simulink model "HSM_4p6U10_Motion_v01_06022022_NEW_ECC_2019a"  (R2019a)
settings: Solver=ode1  StartTime=0.0  StopTime=Inf  FixedStep=Ts  RelTol=1e-3  EnableMultiTasking=on
PostLoadFcn:
  | , if any(exist('dsrtsu_mdlpostloadfcn', 'file') == [2, 3, 6]), try dsrtsu_mdlpostloadfcn('Execute', bdroot); catch fprintf('Error in PostLoadFcn (dsrtsu_mdlpostloadfcn) for model "%s":\n %s\n', bdroot, lasterr); end, end,
values from neighbouring files (symbols this model uses):
  CDP = -1    [Parameters_4p6U10.m]
  CUP = 1    [Parameters_4p6U10.m]
  HDP = 1    [Parameters_4p6U10.m]
  HUP = -1    [Parameters_4p6U10.m]
  K1m = 1.7E-4    (= 0.00017)    [Parameters_4p6U10.m]
  K2m = 7.0E-4    (= 0.0007)    [Parameters_4p6U10.m]
  Ts = 0.0002    [Parameters_4p6U10.m]
undefined symbols (not defined in the file or in its folder): GPTRIP1SEL, GPTRIP2SEL, TZ1, TZ2
libraries: simulink_extras x25, simulink x17, c2837xDlib x11, c2802xlib x2, idelinklib_common x1
(part 3 of 3)

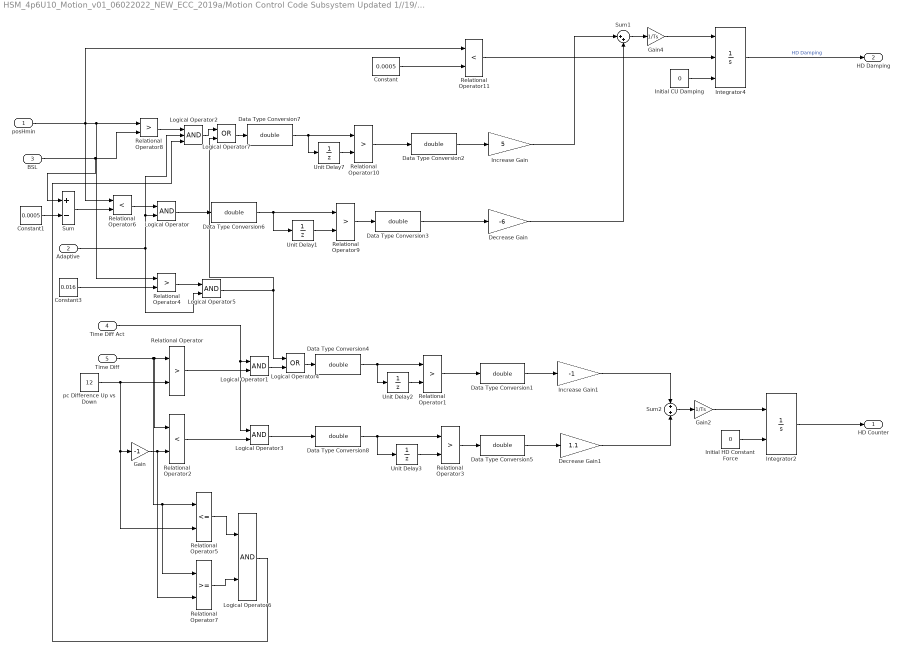
== system HSM_4p6U10_Motion_v01_06022022_NEW_ECC_2019a/Motion Control Code Subsystem Updated 1//19//21/Oscillation, Start Motion, 4 Phases Subsystem/Oscillations Subsystem Time pc No Cold Damping/Subsystem/Approximate Resonance Actuation/Subsystem ==
  posHmin : Inport
  Adaptive : Inport  Port=2
  BSL : Inport  Port=3
  Time Diff Act : Inport  Port=4
  Time Diff : Inport  Port=5
  Constant : Constant  Value=0.0005
  Constant1 : Constant  Value=0.0005
  Constant3 : Constant  Value=0.016
  Data Type Conversion{1..8} (8 alike) : DataTypeConversion  OutDataTypeStr=double
  Decrease Gain : Gain  Gain=-6  OutDataTypeStr=double
  Decrease Gain1 : Gain  Gain=1.1  OutDataTypeStr=double
  Gain : Gain  Gain=-1
  Gain2 : Gain  Gain=1/Ts
  Gain4 : Gain  Gain=1/Ts
  Increase Gain : Gain  Gain=5  OutDataTypeStr=double
  Increase Gain1 : Gain  Gain=-1  OutDataTypeStr=double
  Initial CU Damping : Constant  Value=0  OutDataTypeStr=double
  Initial HD Constant Force : Constant  Value=0  OutDataTypeStr=double
  Integrator2 : Integrator  InitialConditionSource=external  LimitOutput=on  UpperSaturationLimit=2000  LowerSaturationLimit=-2000
  Integrator4 : Integrator  ExternalReset=either  InitialConditionSource=external  LimitOutput=on  UpperSaturationLimit=2000  LowerSaturationLimit=0
  Logical Operator{,1,3,5..6} (5 alike) : Logic  AllPortsSameDT=off  OutDataTypeStr=boolean
  Logical Operator2 : Logic  Inputs=3  AllPortsSameDT=off  OutDataTypeStr=boolean
  Logical Operator4 : Logic  Operator=OR  AllPortsSameDT=off  OutDataTypeStr=boolean
  Logical Operator7 : Logic  Operator=OR  AllPortsSameDT=off  OutDataTypeStr=boolean
  Relational Operator{,1,3..4,8..10} (7 alike) : RelationalOperator  Operator=>  OutDataTypeStr=boolean  RndMeth=Simplest
  Relational Operator11 : RelationalOperator  Operator=<  OutDataTypeStr=boolean  RndMeth=Simplest
  Relational Operator2 : RelationalOperator  Operator=<  OutDataTypeStr=boolean  RndMeth=Simplest
  Relational Operator5 : RelationalOperator  Operator=<=  OutDataTypeStr=boolean  RndMeth=Simplest
  Relational Operator6 : RelationalOperator  Operator=<  OutDataTypeStr=boolean  RndMeth=Simplest
  Relational Operator7 : RelationalOperator  OutDataTypeStr=boolean  RndMeth=Simplest
  Sum : Sum  Inputs=+-
  Sum1 : Sum  Inputs=|++
  Sum2 : Sum
  Unit Delay{1..3,7} (4 alike) : UnitDelay  SampleTime=-1  HasFrameUpgradeWarning=on
  pc Difference Up vs Down : Constant  Value=12
  "HD Counter " : Outport
  HD Damping : Outport  Port=2
  wires:
  BSL/1 -> Relational Operator8/2, Sum/1
  Relational Operator8/1 -> Logical Operator2/1
  Initial CU Damping/1 -> Integrator4/3
  Data Type Conversion6/1 -> Unit Delay1/1, Relational Operator9/1
  Gain4/1 -> Integrator4/1
  Integrator2/1 -> "HD Counter "/1
  Increase Gain/1 -> Sum1/1
  Integrator4/1 -> HD Damping/1  "HD Damping"
  Data Type Conversion7/1 -> Relational Operator10/1, Unit Delay7/1
  Relational Operator10/1 -> Data Type Conversion2/1
  Sum1/1 -> Gain4/1
  posHmin/1 -> Relational Operator6/1, Relational Operator11/1, Relational Operator4/1, Relational Operator8/1
  Logical Operator2/1 -> Logical Operator7/1
  Decrease Gain1/1 -> Sum2/2
  Logical Operator/1 -> Data Type Conversion6/1
  Data Type Conversion2/1 -> Increase Gain/1
  Constant/1 -> Relational Operator11/2
  Unit Delay1/1 -> Relational Operator9/2
  Relational Operator6/1 -> Logical Operator/1
  Sum2/1 -> Gain2/1
  Relational Operator11/1 -> Integrator4/2
  Data Type Conversion3/1 -> Decrease Gain/1
  Increase Gain1/1 -> Sum2/1
  Constant1/1 -> Sum/2
  Adaptive/1 -> Logical Operator2/2, Logical Operator/2, Logical Operator5/2
  Unit Delay7/1 -> Relational Operator10/2
  Sum/1 -> Relational Operator6/2
  Gain2/1 -> Integrator2/1
  Initial HD Constant Force/1 -> Integrator2/2
  Relational Operator9/1 -> Data Type Conversion3/1
  Decrease Gain/1 -> Sum1/2
  Time Diff/1 -> Relational Operator5/1, Relational Operator7/1, Relational Operator2/1, Relational Operator/1
  pc Difference Up vs Down/1 -> Relational Operator/2, Gain/1, Relational Operator5/2
  Relational Operator/1 -> Logical Operator1/2
  Time Diff Act/1 -> Logical Operator1/1, Logical Operator3/1
  Unit Delay2/1 -> Relational Operator1/2
  Data Type Conversion1/1 -> Increase Gain1/1
  Relational Operator1/1 -> Data Type Conversion1/1
  Data Type Conversion4/1 -> Unit Delay2/1, Relational Operator1/1
  Logical Operator1/1 -> Logical Operator4/2
  Gain/1 -> Relational Operator7/2, Relational Operator2/2
  Relational Operator2/1 -> Logical Operator3/2
  Relational Operator3/1 -> Data Type Conversion5/1
  Data Type Conversion5/1 -> Decrease Gain1/1
  Unit Delay3/1 -> Relational Operator3/2
  Data Type Conversion8/1 -> Relational Operator3/1, Unit Delay3/1
  Logical Operator3/1 -> Data Type Conversion8/1
  Logical Operator4/1 -> Data Type Conversion4/1
  Relational Operator4/1 -> Logical Operator5/1
  Constant3/1 -> Relational Operator4/2
  Logical Operator5/1 -> Logical Operator7/2, Logical Operator4/1
  Relational Operator5/1 -> Logical Operator6/1
  Relational Operator7/1 -> Logical Operator6/2
  Logical Operator6/1 -> Logical Operator2/3
  Logical Operator7/1 -> Data Type Conversion7/1

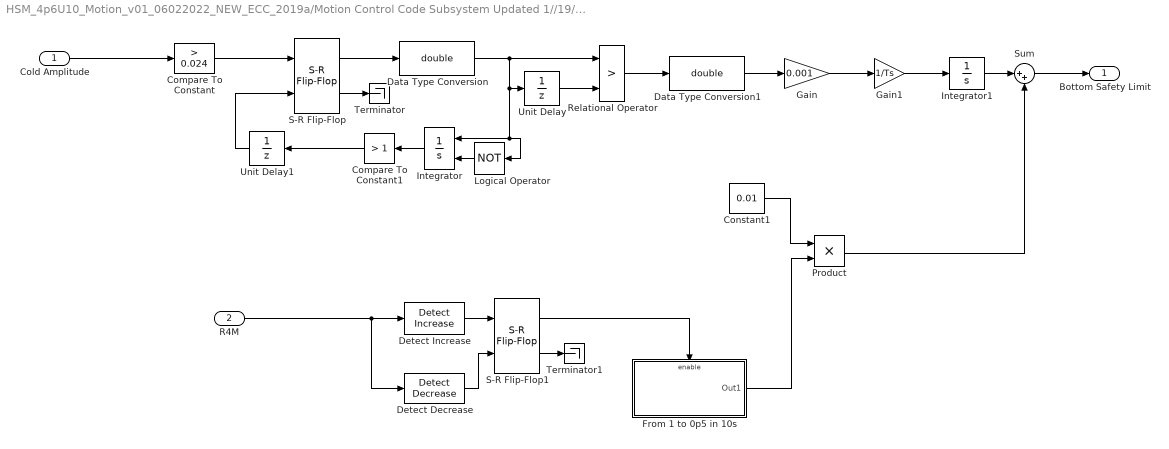
== system HSM_4p6U10_Motion_v01_06022022_NEW_ECC_2019a/Motion Control Code Subsystem Updated 1//19//21/Oscillation, Start Motion, 4 Phases Subsystem/Oscillations Subsystem Time pc No Cold Damping/Subsystem/Approximate Resonance Actuation/Subsystem1 ==
  Cold Amplitude : Inport
  R4M : Inport  Port=2
  Compare To Constant : simulink/Logic and Bit Operations/Compare To Constant  relop=>  const=0.024  OutDataTypeStr=boolean
  Compare To Constant1 : simulink/Logic and Bit Operations/Compare To Constant  relop=>  const=1  OutDataTypeStr=boolean
  Constant1 : Constant  Value=0.01
  Data Type Conversion : DataTypeConversion  OutDataTypeStr=double
  Data Type Conversion1 : DataTypeConversion  OutDataTypeStr=double
  Detect Decrease : simulink/Logic and Bit Operations/Detect Decrease  vinit=0.0  OutDataTypeStr=boolean
  Detect Increase : simulink/Logic and Bit Operations/Detect Increase  vinit=0.0  OutDataTypeStr=boolean
  From 1 to 0p5 in 10s : Subsystem
  Gain : Gain  Gain=0.001
  Gain1 : Gain  Gain=1/Ts
  Integrator : Integrator  ExternalReset=rising
  Integrator1 : Integrator  LimitOutput=on  UpperSaturationLimit=0.006  LowerSaturationLimit=0
  Logical Operator : Logic  Operator=NOT  AllPortsSameDT=off  OutDataTypeStr=boolean
  Product : Product
  Relational Operator : RelationalOperator  Operator=>  OutDataTypeStr=boolean  RndMeth=Simplest
  S-R Flip-Flop : simulink_extras/Flip Flops/S-R Flip-Flop  initial_condition=0
  S-R Flip-Flop1 : simulink_extras/Flip Flops/S-R Flip-Flop  initial_condition=0
  Sum : Sum  Inputs=|++
  Terminator : Terminator
  Terminator1 : Terminator
  Unit Delay : UnitDelay  SampleTime=-1  HasFrameUpgradeWarning=on
  Unit Delay1 : UnitDelay  SampleTime=-1  HasFrameUpgradeWarning=on
  Bottom Safety Limit : Outport
  wires:
  Sum/1 -> Bottom Safety Limit/1
  Integrator1/1 -> Sum/1
  Gain1/1 -> Integrator1/1
  Gain/1 -> Gain1/1
  Unit Delay1/1 -> S-R Flip-Flop/2
  Compare To Constant1/1 -> Unit Delay1/1
  Integrator/1 -> Compare To Constant1/1
  Logical Operator/1 -> Integrator/2
  Data Type Conversion1/1 -> Gain/1
  Relational Operator/1 -> Data Type Conversion1/1
  Unit Delay/1 -> Relational Operator/2
  Data Type Conversion/1 -> Relational Operator/1, Unit Delay/1, Integrator/1, Logical Operator/1
  S-R Flip-Flop/1 -> Data Type Conversion/1
  S-R Flip-Flop/2 -> Terminator/1
  Compare To Constant/1 -> S-R Flip-Flop/1
  Cold Amplitude/1 -> Compare To Constant/1
  Product/1 -> Sum/2
  From 1 to 0p5 in 10s/1(Out1) -> Product/2
  S-R Flip-Flop1/2 -> Terminator1/1
  R4M/1 -> Detect Decrease/1, Detect Increase/1
  S-R Flip-Flop1/1 -> From 1 to 0p5 in 10s/Enable
  Detect Decrease/1 -> S-R Flip-Flop1/2
  Detect Increase/1 -> S-R Flip-Flop1/1
  Constant1/1 -> Product/1

== system HSM_4p6U10_Motion_v01_06022022_NEW_ECC_2019a/Motion Control Code Subsystem Updated 1//19//21/Oscillation, Start Motion, 4 Phases Subsystem/Oscillations Subsystem Time pc No Cold Damping/Subsystem/Approximate Resonance Actuation/Subsystem2 ==
  PosH : Inport
  VelH : Inport  Port=2
  Bot Safety Limit : Inport  Port=3
  posHFRTime : Inport  Port=4
  AND1 : Logic  AllPortsSameDT=off  OutDataTypeStr=boolean
  Constant3 : Constant  Value=0
  Constant5 : Constant  Value=0
  HD Act : simulink_extras/Flip Flops/S-R Flip-Flop  initial_condition=0
  Logical Operator1 : Logic  Operator=OR  AllPortsSameDT=off  OutDataTypeStr=boolean
  OR1 : Logic  Operator=OR  AllPortsSameDT=off  OutDataTypeStr=boolean
  Relational Operator5 : RelationalOperator  Operator=<=  OutDataTypeStr=boolean  RndMeth=Simplest
  Relational Operator6 : RelationalOperator  Operator=>  OutDataTypeStr=boolean  RndMeth=Simplest
  Relational Operator8 : RelationalOperator  Operator=<  OutDataTypeStr=boolean  RndMeth=Simplest
  Relational Operator9 : RelationalOperator  Operator=<  OutDataTypeStr=boolean  RndMeth=Simplest
  Start Hot Down : Constant  Value=0.035
  Subsystem : Subsystem
  Terminator : Terminator
  Unit Delay : UnitDelay  SampleTime=-1  HasFrameUpgradeWarning=on
  HD Activation : Outport
  wires:
  Unit Delay/1 -> HD Act/2
  Logical Operator1/1 -> Unit Delay/1
  HD Act/2 -> Terminator/1
  HD Act/1 -> Subsystem/2(Q Boolean), HD Activation/1  "HD Act"
  Relational Operator6/1 -> OR1/2  "VelH > 0"
  Constant3/1 -> Relational Operator6/2
  Relational Operator5/1 -> OR1/1  "PosH <= Bot Safety"
  Bot Safety Limit/1 -> Relational Operator5/2
  PosH/1 -> Subsystem/3(posH), Relational Operator8/1, Relational Operator5/1
  Constant5/1 -> Relational Operator9/2
  Relational Operator9/1 -> AND1/2  "VelH   < 0"
  Relational Operator8/1 -> AND1/1  "PosH  < 0.025"
  AND1/1 -> HD Act/1
  Start Hot Down/1 -> Relational Operator8/2
  VelH/1 -> Relational Operator9/1, Relational Operator6/1
  OR1/1 -> Logical Operator1/1
  posHFRTime/1 -> Subsystem/1(posHFRTime)
  Subsystem/1(Reset) -> Logical Operator1/2

== system HSM_4p6U10_Motion_v01_06022022_NEW_ECC_2019a/Motion Control Code Subsystem Updated 1//19//21/Oscillation, Start Motion, 4 Phases Subsystem/Oscillations Subsystem Time pc No Cold Damping/Subsystem/Hot Down Control/Unity Gain Scaling ==
  u : Inport
  x : Inport  Port=2
  Constant6 : Constant  Value=K2m
  Gain1 : Gain  Gain=-1/K1m
  IYC Saturation : Saturate  UpperLimit=3600  LowerLimit=0
  Math Function4 : Math  Operator=square  SaturateOnIntegerOverflow=on
  Product1 : Product
  Sqrt : Sqrt  SaturateOnIntegerOverflow=on
  Sum3 : Sum
  i : Outport
  wires:
  IYC Saturation/1 -> Sqrt/1
  Sqrt/1 -> i/1
  Product1/1 -> IYC Saturation/1
  Gain1/1 -> Product1/1
  x/1 -> Sum3/2
  Math Function4/1 -> Product1/2
  Constant6/1 -> Sum3/1
  Sum3/1 -> Math Function4/1
  u/1 -> Gain1/1

== system HSM_4p6U10_Motion_v01_06022022_NEW_ECC_2019a/Motion Control Code Subsystem Updated 1//19//21/Oscillation, Start Motion, 4 Phases Subsystem/Oscillations Subsystem Time pc No Cold Damping/Cold Resonance/Approximate Resonance Actuation/CD Damping/Subsystem ==
  In1 : Inport
  Data Type Conversion1 : DataTypeConversion  OutDataTypeStr=double
  Data Type Conversion2 : DataTypeConversion  OutDataTypeStr=double
  Relational Operator4 : RelationalOperator  Operator=>  OutDataTypeStr=boolean  RndMeth=Simplest
  Unit Delay2 : UnitDelay  SampleTime=-1  HasFrameUpgradeWarning=on
  Out1 : Outport
  wires:
  Relational Operator4/1 -> Data Type Conversion2/1
  Data Type Conversion2/1 -> Out1/1
  Data Type Conversion1/1 -> Relational Operator4/1, Unit Delay2/1
  Unit Delay2/1 -> Relational Operator4/2
  In1/1 -> Data Type Conversion1/1

== system HSM_4p6U10_Motion_v01_06022022_NEW_ECC_2019a/Motion Control Code Subsystem Updated 1//19//21/Oscillation, Start Motion, 4 Phases Subsystem/Oscillations Subsystem Time pc No Cold Damping/Cold Resonance/Approximate Resonance Actuation/CD Damping/Subsystem1 ==
  In1 : Inport
  Data Type Conversion3 : DataTypeConversion  OutDataTypeStr=double
  Data Type Conversion4 : DataTypeConversion  OutDataTypeStr=double
  Relational Operator5 : RelationalOperator  Operator=>  OutDataTypeStr=boolean  RndMeth=Simplest
  Unit Delay1 : UnitDelay  SampleTime=-1  HasFrameUpgradeWarning=on
  Out1 : Outport
  wires:
  Data Type Conversion4/1 -> Out1/1
  Unit Delay1/1 -> Relational Operator5/2
  Relational Operator5/1 -> Data Type Conversion4/1
  In1/1 -> Data Type Conversion3/1
  Data Type Conversion3/1 -> Unit Delay1/1, Relational Operator5/1

== system HSM_4p6U10_Motion_v01_06022022_NEW_ECC_2019a/Motion Control Code Subsystem Updated 1//19//21/Oscillation, Start Motion, 4 Phases Subsystem/Oscillations Subsystem Time pc No Cold Damping/Cold Resonance/Approximate Resonance Actuation/CD Damping/Subsystem2 ==
  In1 : Inport
  Data Type Conversion3 : DataTypeConversion  OutDataTypeStr=double
  Data Type Conversion4 : DataTypeConversion  OutDataTypeStr=double
  Relational Operator5 : RelationalOperator  Operator=>  OutDataTypeStr=boolean  RndMeth=Simplest
  Unit Delay1 : UnitDelay  SampleTime=-1  HasFrameUpgradeWarning=on
  Out1 : Outport
  wires:
  Data Type Conversion3/1 -> Relational Operator5/1, Unit Delay1/1
  In1/1 -> Data Type Conversion3/1
  Relational Operator5/1 -> Data Type Conversion4/1
  Unit Delay1/1 -> Relational Operator5/2
  Data Type Conversion4/1 -> Out1/1

== system HSM_4p6U10_Motion_v01_06022022_NEW_ECC_2019a/Motion Control Code Subsystem Updated 1//19//21/Oscillation, Start Motion, 4 Phases Subsystem/Oscillations Subsystem Time pc No Cold Damping/Cold Resonance/Approximate Resonance Actuation/CD Damping/Subsystem3 ==
  In1 : Inport
  Data Type Conversion3 : DataTypeConversion  OutDataTypeStr=double
  Data Type Conversion4 : DataTypeConversion  OutDataTypeStr=double
  Relational Operator5 : RelationalOperator  Operator=>  OutDataTypeStr=boolean  RndMeth=Simplest
  Unit Delay1 : UnitDelay  SampleTime=-1  HasFrameUpgradeWarning=on
  Out1 : Outport
  wires:
  Data Type Conversion4/1 -> Out1/1
  Unit Delay1/1 -> Relational Operator5/2
  Relational Operator5/1 -> Data Type Conversion4/1
  In1/1 -> Data Type Conversion3/1
  Data Type Conversion3/1 -> Unit Delay1/1, Relational Operator5/1

== system HSM_4p6U10_Motion_v01_06022022_NEW_ECC_2019a/Motion Control Code Subsystem Updated 1//19//21/Oscillation, Start Motion, 4 Phases Subsystem/Oscillations Subsystem Time pc No Cold Damping/Cold Resonance/Approximate Resonance Actuation/CD Damping/Subsystem4 ==
  In1 : Inport
  Data Type Conversion3 : DataTypeConversion  OutDataTypeStr=double
  Data Type Conversion4 : DataTypeConversion  OutDataTypeStr=double
  Relational Operator5 : RelationalOperator  Operator=>  OutDataTypeStr=boolean  RndMeth=Simplest
  Unit Delay1 : UnitDelay  SampleTime=-1  HasFrameUpgradeWarning=on
  Out1 : Outport
  wires:
  Data Type Conversion4/1 -> Out1/1
  Unit Delay1/1 -> Relational Operator5/2
  Relational Operator5/1 -> Data Type Conversion4/1
  In1/1 -> Data Type Conversion3/1
  Data Type Conversion3/1 -> Unit Delay1/1, Relational Operator5/1

== system HSM_4p6U10_Motion_v01_06022022_NEW_ECC_2019a/Motion Control Code Subsystem Updated 1//19//21/Oscillation, Start Motion, 4 Phases Subsystem/Oscillations Subsystem Time pc No Cold Damping/Cold Resonance/Approximate Resonance Actuation/CD Damping/Subsystem5 ==
  In1 : Inport
  Data Type Conversion3 : DataTypeConversion  OutDataTypeStr=double
  Data Type Conversion4 : DataTypeConversion  OutDataTypeStr=double
  Relational Operator5 : RelationalOperator  Operator=>  OutDataTypeStr=boolean  RndMeth=Simplest
  Unit Delay1 : UnitDelay  SampleTime=-1  HasFrameUpgradeWarning=on
  Out1 : Outport
  wires:
  Data Type Conversion3/1 -> Relational Operator5/1, Unit Delay1/1
  In1/1 -> Data Type Conversion3/1
  Relational Operator5/1 -> Data Type Conversion4/1
  Unit Delay1/1 -> Relational Operator5/2
  Data Type Conversion4/1 -> Out1/1

== system HSM_4p6U10_Motion_v01_06022022_NEW_ECC_2019a/Motion Control Code Subsystem Updated 1//19//21/Oscillation, Start Motion, 4 Phases Subsystem/Oscillations Subsystem Time pc No Cold Damping/Cold Resonance/Approximate Resonance Actuation/CU Damping/Subsystem ==
  In1 : Inport
  Data Type Conversion1 : DataTypeConversion  OutDataTypeStr=double
  Data Type Conversion2 : DataTypeConversion  OutDataTypeStr=double
  Relational Operator4 : RelationalOperator  Operator=>  OutDataTypeStr=boolean  RndMeth=Simplest
  Unit Delay2 : UnitDelay  SampleTime=-1  HasFrameUpgradeWarning=on
  Out1 : Outport
  wires:
  In1/1 -> Data Type Conversion1/1
  Unit Delay2/1 -> Relational Operator4/2
  Data Type Conversion1/1 -> Unit Delay2/1, Relational Operator4/1
  Data Type Conversion2/1 -> Out1/1
  Relational Operator4/1 -> Data Type Conversion2/1

== system HSM_4p6U10_Motion_v01_06022022_NEW_ECC_2019a/Motion Control Code Subsystem Updated 1//19//21/Oscillation, Start Motion, 4 Phases Subsystem/Oscillations Subsystem Time pc No Cold Damping/Cold Resonance/Approximate Resonance Actuation/CU Damping/Subsystem1 ==
  In1 : Inport
  Data Type Conversion3 : DataTypeConversion  OutDataTypeStr=double
  Data Type Conversion4 : DataTypeConversion  OutDataTypeStr=double
  Relational Operator5 : RelationalOperator  Operator=>  OutDataTypeStr=boolean  RndMeth=Simplest
  Unit Delay1 : UnitDelay  SampleTime=-1  HasFrameUpgradeWarning=on
  Out1 : Outport
  wires:
  Data Type Conversion3/1 -> Relational Operator5/1, Unit Delay1/1
  In1/1 -> Data Type Conversion3/1
  Relational Operator5/1 -> Data Type Conversion4/1
  Unit Delay1/1 -> Relational Operator5/2
  Data Type Conversion4/1 -> Out1/1

== system HSM_4p6U10_Motion_v01_06022022_NEW_ECC_2019a/Motion Control Code Subsystem Updated 1//19//21/Oscillation, Start Motion, 4 Phases Subsystem/Oscillations Subsystem Time pc No Cold Damping/Cold Resonance/Approximate Resonance Actuation/CU Damping/Subsystem2 ==
  In1 : Inport
  Data Type Conversion3 : DataTypeConversion  OutDataTypeStr=double
  Data Type Conversion4 : DataTypeConversion  OutDataTypeStr=double
  Relational Operator5 : RelationalOperator  Operator=>  OutDataTypeStr=boolean  RndMeth=Simplest
  Unit Delay1 : UnitDelay  SampleTime=-1  HasFrameUpgradeWarning=on
  Out1 : Outport
  wires:
  Data Type Conversion4/1 -> Out1/1
  Unit Delay1/1 -> Relational Operator5/2
  Relational Operator5/1 -> Data Type Conversion4/1
  In1/1 -> Data Type Conversion3/1
  Data Type Conversion3/1 -> Unit Delay1/1, Relational Operator5/1

== system HSM_4p6U10_Motion_v01_06022022_NEW_ECC_2019a/Motion Control Code Subsystem Updated 1//19//21/Oscillation, Start Motion, 4 Phases Subsystem/Oscillations Subsystem Time pc No Cold Damping/Cold Resonance/Approximate Resonance Actuation/CU Damping/Subsystem3 ==
  In1 : Inport
  Data Type Conversion3 : DataTypeConversion  OutDataTypeStr=double
  Data Type Conversion4 : DataTypeConversion  OutDataTypeStr=double
  Relational Operator5 : RelationalOperator  Operator=>  OutDataTypeStr=boolean  RndMeth=Simplest
  Unit Delay1 : UnitDelay  SampleTime=-1  HasFrameUpgradeWarning=on
  Out1 : Outport
  wires:
  Data Type Conversion3/1 -> Relational Operator5/1, Unit Delay1/1
  In1/1 -> Data Type Conversion3/1
  Relational Operator5/1 -> Data Type Conversion4/1
  Unit Delay1/1 -> Relational Operator5/2
  Data Type Conversion4/1 -> Out1/1

== system HSM_4p6U10_Motion_v01_06022022_NEW_ECC_2019a/Motion Control Code Subsystem Updated 1//19//21/Oscillation, Start Motion, 4 Phases Subsystem/Oscillations Subsystem Time pc No Cold Damping/Cold Resonance/Approximate Resonance Actuation/CU Damping/Subsystem4 ==
  In1 : Inport
  Data Type Conversion3 : DataTypeConversion  OutDataTypeStr=double
  Data Type Conversion4 : DataTypeConversion  OutDataTypeStr=double
  Relational Operator5 : RelationalOperator  Operator=>  OutDataTypeStr=boolean  RndMeth=Simplest
  Unit Delay1 : UnitDelay  SampleTime=-1  HasFrameUpgradeWarning=on
  Out1 : Outport
  wires:
  Data Type Conversion3/1 -> Relational Operator5/1, Unit Delay1/1
  In1/1 -> Data Type Conversion3/1
  Relational Operator5/1 -> Data Type Conversion4/1
  Unit Delay1/1 -> Relational Operator5/2
  Data Type Conversion4/1 -> Out1/1

== system HSM_4p6U10_Motion_v01_06022022_NEW_ECC_2019a/Motion Control Code Subsystem Updated 1//19//21/Oscillation, Start Motion, 4 Phases Subsystem/Oscillations Subsystem Time pc No Cold Damping/Cold Resonance/Approximate Resonance Actuation/CU Damping/Subsystem5 ==
  In1 : Inport
  Data Type Conversion3 : DataTypeConversion  OutDataTypeStr=double
  Data Type Conversion4 : DataTypeConversion  OutDataTypeStr=double
  Relational Operator5 : RelationalOperator  Operator=>  OutDataTypeStr=boolean  RndMeth=Simplest
  Unit Delay1 : UnitDelay  SampleTime=-1  HasFrameUpgradeWarning=on
  Out1 : Outport
  wires:
  Data Type Conversion4/1 -> Out1/1
  Unit Delay1/1 -> Relational Operator5/2
  Relational Operator5/1 -> Data Type Conversion4/1
  In1/1 -> Data Type Conversion3/1
  Data Type Conversion3/1 -> Unit Delay1/1, Relational Operator5/1

== system HSM_4p6U10_Motion_v01_06022022_NEW_ECC_2019a/Motion Control Code Subsystem Updated 1//19//21/Oscillation, Start Motion, 4 Phases Subsystem/Oscillations Subsystem Time pc No Cold Damping/Cold Resonance/Approximate Resonance Actuation/Calculate Cold Amp and Bias/Grab Max Position Option 1 ==
  Position : Inport
  Enable : EnablePort  StatesWhenEnabling=reset
  Max Position : Outport
  wires:
  Position/1 -> Max Position/1  "Max Position"

== system HSM_4p6U10_Motion_v01_06022022_NEW_ECC_2019a/Motion Control Code Subsystem Updated 1//19//21/Oscillation, Start Motion, 4 Phases Subsystem/Oscillations Subsystem Time pc No Cold Damping/Cold Resonance/Approximate Resonance Actuation/Calculate Cold Amp and Bias/Grab Max Position Option 2 ==
  Position : Inport
  Enable : EnablePort  StatesWhenEnabling=reset
  Max Position : Outport
  wires:
  Position/1 -> Max Position/1  "Max Position"

== system HSM_4p6U10_Motion_v01_06022022_NEW_ECC_2019a/Motion Control Code Subsystem Updated 1//19//21/Oscillation, Start Motion, 4 Phases Subsystem/Oscillations Subsystem Time pc No Cold Damping/Cold Resonance/Approximate Resonance Actuation/Calculate Cold Amp and Bias/Subsystem ==
  Max : Inport
  Min : Inport  Port=2
  Enable : EnablePort
  Gain : Gain  Gain=1/2
  Sum : Sum
  Sum1 : Sum  Inputs=+-
  Bias : Outport
  Cold Amplitude : Outport  Port=2
  wires:
  Sum1/1 -> Cold Amplitude/1
  Gain/1 -> Bias/1, Sum1/2  "Bias"
  Sum/1 -> Gain/1
  Min/1 -> Sum/2
  Max/1 -> Sum/1, Sum1/1

== system HSM_4p6U10_Motion_v01_06022022_NEW_ECC_2019a/Motion Control Code Subsystem Updated 1//19//21/Oscillation, Start Motion, 4 Phases Subsystem/Oscillations Subsystem Time pc No Cold Damping/Cold Resonance/Approximate Resonance Actuation/Calculate Cold Amp and Bias/Subsystem1 ==
  velC : Inport
  Constant1 : Constant  Value=0  OutDataTypeStr=boolean
  Logical Operator : Logic  AllPortsSameDT=off  OutDataTypeStr=boolean
  Relational Operator1 : RelationalOperator  Operator=>  OutDataTypeStr=boolean  RndMeth=Simplest
  Relational Operator2 : RelationalOperator  Operator=<=  OutDataTypeStr=boolean  RndMeth=Simplest
  Unit Delay1 : UnitDelay  SampleTime=-1  HasFrameUpgradeWarning=on
  velC Cross : Outport
  wires:
  velC/1 -> Unit Delay1/1, Relational Operator2/1
  Logical Operator/1 -> velC Cross/1
  Constant1/1 -> Relational Operator1/2, Relational Operator2/2
  Unit Delay1/1 -> Relational Operator1/1
  Relational Operator2/1 -> Logical Operator/2
  Relational Operator1/1 -> Logical Operator/1

== system HSM_4p6U10_Motion_v01_06022022_NEW_ECC_2019a/Motion Control Code Subsystem Updated 1//19//21/Oscillation, Start Motion, 4 Phases Subsystem/Oscillations Subsystem Time pc No Cold Damping/Cold Resonance/Approximate Resonance Actuation/Calculate Cold Amp and Bias/Subsystem2 ==
  velC : Inport
  Constant2 : Constant  Value=0  OutDataTypeStr=boolean
  Logical Operator2 : Logic  AllPortsSameDT=off  OutDataTypeStr=boolean
  Relational Operator4 : RelationalOperator  Operator=<  OutDataTypeStr=boolean  RndMeth=Simplest
  Relational Operator5 : RelationalOperator  OutDataTypeStr=boolean  RndMeth=Simplest
  Unit Delay4 : UnitDelay  SampleTime=-1  HasFrameUpgradeWarning=on
  velC Cross : Outport
  wires:
  Relational Operator4/1 -> Logical Operator2/1
  Constant2/1 -> Relational Operator5/2, Relational Operator4/2
  Logical Operator2/1 -> velC Cross/1
  Unit Delay4/1 -> Relational Operator4/1
  Relational Operator5/1 -> Logical Operator2/2
  velC/1 -> Relational Operator5/1, Unit Delay4/1

== system HSM_4p6U10_Motion_v01_06022022_NEW_ECC_2019a/Motion Control Code Subsystem Updated 1//19//21/Oscillation, Start Motion, 4 Phases Subsystem/Oscillations Subsystem Time pc No Cold Damping/Subsystem/Approximate Resonance Actuation/Subsystem1/From 1 to 0p5 in 10s ==
  Enable : EnablePort  StatesWhenEnabling=reset
  Constant : Constant
  Gain : Gain  Gain=-0.05
  Integrator : Integrator  LimitOutput=on  UpperSaturationLimit=20  LowerSaturationLimit=0
  Limit Saturation : Saturate  UpperLimit=1  LowerLimit=0.5
  Sum : Sum  Inputs=|++
  Unit : Constant
  Out1 : Outport
  wires:
  Limit Saturation/1 -> Out1/1
  Sum/1 -> Limit Saturation/1
  Unit/1 -> Sum/2
  Gain/1 -> Sum/1
  Integrator/1 -> Gain/1
  Constant/1 -> Integrator/1

== system HSM_4p6U10_Motion_v01_06022022_NEW_ECC_2019a/Motion Control Code Subsystem Updated 1//19//21/Oscillation, Start Motion, 4 Phases Subsystem/Oscillations Subsystem Time pc No Cold Damping/Subsystem/Approximate Resonance Actuation/Subsystem2/Subsystem ==
  posHFRTime : Inport
  Q Boolean : Inport  Port=2
  posH : Inport  Port=3
  Compare To Constant : simulink/Logic and Bit Operations/Compare To Constant  relop=>  const=0  OutDataTypeStr=boolean
  Constant1 : Constant  Value=0.018
  Data Type Conversion : DataTypeConversion  OutDataTypeStr=double
  Hit Crossing : HitCross  HitCrossingOffset=0.025  HitCrossingDirection=rising
  Integrator : Integrator  ExternalReset=rising
  Logical Operator : Logic  AllPortsSameDT=off  OutDataTypeStr=boolean
  Logical Operator2 : Logic  Inputs=3  AllPortsSameDT=off  OutDataTypeStr=boolean
  Relational Operator : RelationalOperator  OutDataTypeStr=boolean  RndMeth=Simplest
  Relational Operator1 : RelationalOperator  Operator=<  OutDataTypeStr=boolean  RndMeth=Simplest
  Reset : Outport
  wires:
  Relational Operator1/1 -> Logical Operator2/3
  Data Type Conversion/1 -> Integrator/1
  Compare To Constant/1 -> Logical Operator/1, Logical Operator2/1
  Constant1/1 -> Relational Operator1/2
  Integrator/1 -> Relational Operator/1
  Relational Operator/1 -> Logical Operator2/2
  Logical Operator2/1 -> Reset/1
  posHFRTime/1 -> Relational Operator/2, Compare To Constant/1
  Logical Operator/1 -> Data Type Conversion/1
  posH/1 -> Hit Crossing/1, Relational Operator1/1
  Hit Crossing/1 -> Integrator/2
  Q Boolean/1 -> Logical Operator/2
